simulink model "MotorSlider_Sim_IFT"  (R2026a)
settings: Solver=VariableStepAuto  StopTime=2.5
settings Model: Creator=lin-t  LastModifiedBy=adam
settings SimscapeCC: SimscapeNominalValues="[{\"value\":\"1\",\"unit\":\"A\"},{\"value\":\"1\",\"unit\":\"bar\"},{\"value\":\"1\",\"unit\":\"cm^2\"},{\"value\":\"1\",\"unit\":\"cm^3/s\"},{\"value\":\"1\",\"unit\":\"kJ/kg\"},{\"value\":\"1\",\"unit\":\"kW\"},{\"value\":\"1\",\"unit\":\"l\"},{\"value\":\"1\",\"unit\":\"N\"},{\"value\":\"1\",\"unit\":\"N*m\"},{\"value\":\"1\",\"unit\":\"V\"}]"  SimscapeLogType=none  SimscapeLogDataHistory=5000.0

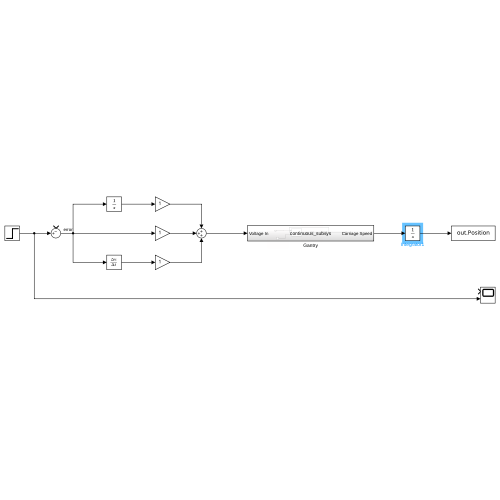
[thumbnail: Simulink's stored preview of the top-level diagram]
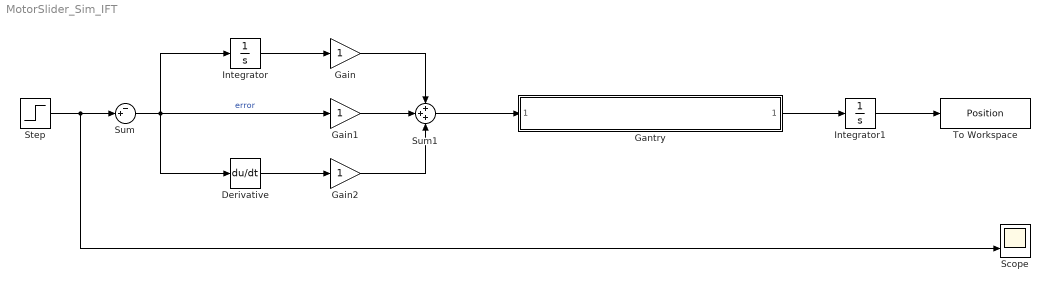
== system MotorSlider_Sim_IFT ==
  Derivative : Derivative
  Gain : Gain
  Gain1 : Gain
  Gain2 : Gain
  Gantry : Subsystem  ReferencedSubsystem=continuous_subsys
  Integrator : Integrator
  Integrator1 : Integrator
  Scope : Scope  NumInputPorts=2
      settings: ActiveDisplayYMinimum=-1.3760095539481985  ActiveDisplayYMaximum=2.649003689371205
  Step : Step  FinalValue=2  SampleTime=0.015
  Sum : Sum  Inputs=-+|
  Sum1 : Sum  Inputs=+++
  To Workspace : ToWorkspace  VariableName=Position  SaveFormat=Timeseries  SampleTime=0.015
  wires:
  Step/1 -> Scope/2, Sum/2
  Sum/1 -> Derivative/1, Gain1/1, Integrator/1  "error"
  Sum1/1 -> Gantry/1
  Integrator/1 -> Gain/1
  Derivative/1 -> Gain2/1
  Gain1/1 -> Sum1/2
  Gain/1 -> Sum1/1
  Gain2/1 -> Sum1/3
  Gantry/1 -> Integrator1/1
  Integrator1/1 -> To Workspace/1
